simulink model "nlmpc_simulink"  (R2023a)
settings: Solver=VariableStepAuto  StartTime=0.0  StopTime=inf  RelTol=1e-3
settings Model: Creator=pindiche  LastModifiedBy=pindiche

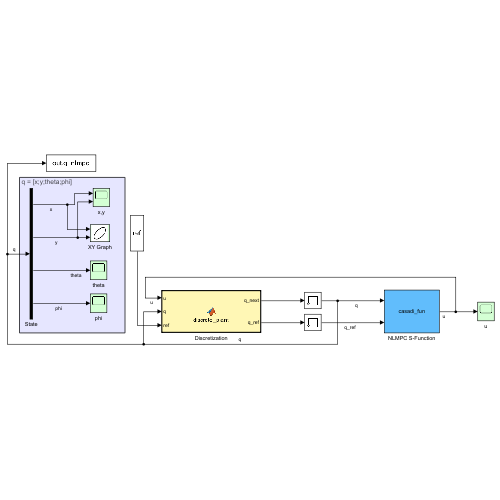
[thumbnail: Simulink's stored preview of the top-level diagram]
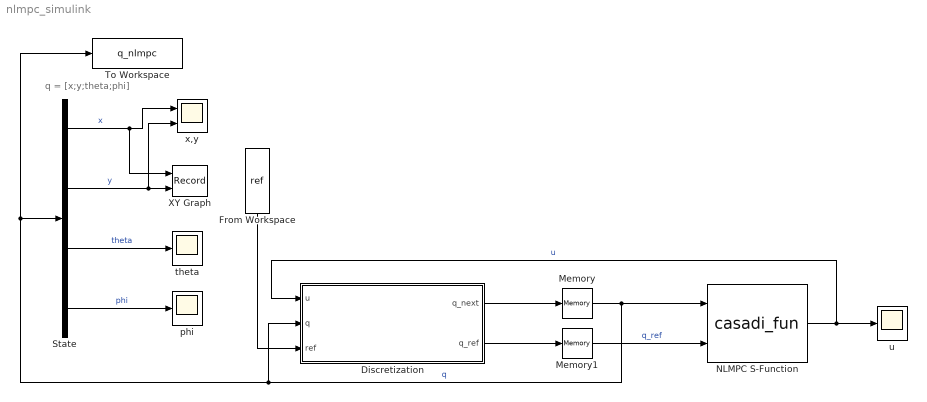
== system nlmpc_simulink ==
  note: q = [x;y;theta;phi]
  Discretization : MATLAB Function  TreatAsAtomicUnit=on
  From Workspace : FromWorkspace  VariableName=ref  SampleTime=0.1  ZeroCross=off
  Memory : Memory
  Memory1 : Memory
  NLMPC S-Function : S-Function  FunctionName=casadi_fun  Parameters='mpc_fun.casadi','mpc_fun'  SFunctionDeploymentMode=off  EnableBusSupport=off
  State : Demux
  To Workspace : ToWorkspace  VariableName=q_nlmpc  SaveFormat=Timeseries  SampleTime=-1
  XY Graph : Record  FileSettingsInternal="{\"entries\":[{\"content\":{\"excelSettings\":{\"content\":{},\"type\":\"Streamout.ExcelSettings\"}},\"type\":\"Streamout.FileSettingStorage\",\"uuid\":\"\"}],\"packageUris\":[\"http:\\/\\/schema.mathworks.com\\/mf0\\/streamout_blocks\\/R2020a\"],\"version\":\"1.0\"}"  Layout=[1 1]  SignalsInternal="{\"entries\":[{\"content\":{\"signals\":[{\"content\":{\"blockPath\":[],\"dimensions\":[1,1],\"domain\":\"\",\"lineColor\":\"#a2142f\",\"plots\":[1],\"port\":1,\"sid\":[\"\"],\"signalID\":8923,\"signalName\":\"x\"},\"type\":\"RecordBlkView.Signal\",\"uuid\":\"\"},{\"content\":{\"blockPath\":[],\"dimensions\":[1,1],\"domain\":\"\",\"lineColor\":\"#139fff\",\"plots\":[1],\"port\":2,\"sid\":[\"\"],\"signalID\":8927,\"signalName\":\"y\"},\"type\":\"RecordBlkView.Signal\",\"uuid\":\"\"}]},\"type\":\"RecordBlkView.InputSignals\",\"uuid\":\"\"}],\"packageUris\":[\"http:\\/\\/schema.mathworks.com\\/mf0\\/streamout_blocks\\/R2020a\"],\"version\":\"1.0\"}"  VisualizationBindings="{\"xyplotplugin\":{\"info\":[{\"series\":[{\"bindingParametersList\":[{\"parameter\":\"X-Axis\",\"signalID\":8923,\"signalName\":\"x\"},{\"parameter\":\"Y-Axis\",\"signalID\":8927,\"signalName\":\"y\"}],\"seriesID\":27118}],\"subplotID\":1}]}}"  CompatibilityTag=XY
  phi : Scope
  theta : Scope
  u : Scope
  x,y : Scope  NumInputPorts=2
  wires:
  NLMPC S-Function/1 -> Discretization/1(u), u/1  "u"
  State/4 -> phi/1  "phi"
  State/2 -> x,y/2, XY Graph/2  "y"
  Memory/1 -> Discretization/2(q), To Workspace/1, State/1, NLMPC S-Function/1  "q"
  State/3 -> theta/1  "theta"
  State/1 -> XY Graph/1, x,y/1  "x"
  Memory1/1 -> NLMPC S-Function/2  "q_ref"
  Discretization/1(q_next) -> Memory/1
  Discretization/2(q_ref) -> Memory1/1
  From Workspace/1 -> Discretization/3(ref)

== matlab function nlmpc_simulink/Discretization ==
  data: u input; q_next output; q input; q_ref output; ref input
function [q_next, q_ref] = discrete_plant(u, q, ref)
    persistent idx q_ref_internal;

    if isempty(idx)
        idx = 1;
    end

    if isempty(q_ref_internal)
        q_ref_internal = zeros(4,1);
    end

    % Parameters
    Npred = 12;
    l = 0.256;
    L = l;
    Delta = 0.35;
    dt = 0.1;  
    x = q(1);
    y = q(2);
    theta = q(3);
    phi = q(4);
    
    % Extract control inputs
    v = u(1); 
    omega = u(2);  

    % Discretized system dynamics
    x_next = x + dt * (v * cos(theta));  
    y_next = y + dt * (v * sin(theta)); 
    theta_next = theta + dt * (v / l * tan(phi));  
    phi_next = phi + dt * omega; 
    
    % Reference switching logic
    % if idx == 1
    %     q_ref_internal = [2; 7; pi/2; 0];
    % elseif idx == 40
    %     q_ref_internal = [-1; 2; 0; 0];
    % end

    % q_ref = q_ref_internal;

    % circle
    t = 0:dt:60;  
    % alpha   = 5;
    % beta    = 5;
    % ang     = 0.2;
    % xr = alpha*cos(ang*t);      dxr = -alpha*ang*sin(ang*t);    ddxr = -alpha*ang*ang*cos(ang*t);       dddxr = alpha*ang*ang*ang*sin(ang*t);
    % yr = beta*sin(ang*t);       dyr = beta*ang*cos(ang*t);      ddyr = -beta*ang*ang*sin(ang*t);        dddyr = -beta*ang*ang*ang*cos(ang*t);
    
    % spline
    xr = ref(2);
    yr = ref(3);
    dddxr = ref(4);
    dddyr = ref(5);
    ddxr = ref(6);
    ddyr = ref(7);
    dxr = ref(8);
    dyr = ref(9);

    Vr = sqrt(dxr.^2 + dyr.^2);
    thetar = unwrap(atan2(dyr, dxr));
    phir = atan((l*(ddyr.*dxr - ddxr.*dyr)) ./ Vr.^3);
    
    % references predefined inside here
    % q_ref = zeros(4, Npred + 1);
    % idx_end = min(idx + Npred, size(t,2));

    % q_ref(1, :) = xr(idx:idx_end);
    % q_ref(2, :) = yr(idx:idx_end);
    % q_ref(3, :) = thetar(idx:idx_end);
    % q_ref(4, :) = phir(idx:idx_end);

    q_ref_internal = [xr; yr; thetar; phir];
    q_ref = q_ref_internal;

    q_next = [x_next; y_next; theta_next; phi_next];
    idx = idx + 1;
end
